simulink model "pwm_dc_control"  (R2022a)
settings: Solver=VariableStepAuto  StartTime=0.0  StopTime=4  RelTol=1e-3
model workspace (MATLAB code in the model file):
  | R = 1.71;
  | L = 1.1*10^-4;
  | kT = 5.9*10^-3;
  | kB = 2.75*10^-4;
  | I = 3.88*10^-7;
  | B = [0, -1/I; 1/L, 0];
  | A = [0, kT/I; -kB/L, -R/L];
  | C = [1, 0];
libraries: simulink x2
settings Model: Creator=ba13  LastModifiedBy=ba13
settings DataIOCC: Refine=100

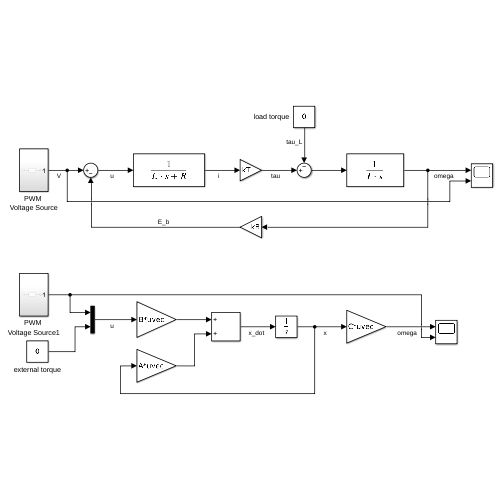
[thumbnail: Simulink's stored preview of the top-level diagram]
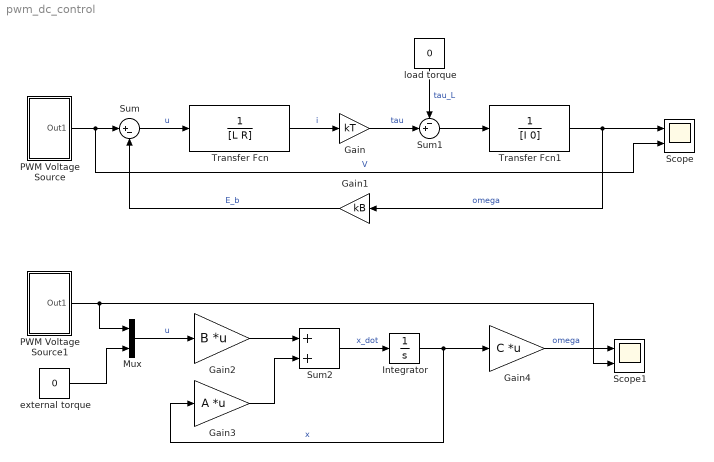
== system pwm_dc_control ==
  Gain : Gain  Gain=kT
  Gain1 : Gain  Gain=kB
  Gain2 : Gain  Gain=B  Multiplication=Matrix(K*u) (u vector)
  Gain3 : Gain  Gain=A  Multiplication=Matrix(K*u) (u vector)
  Gain4 : Gain  Gain=C  Multiplication=Matrix(K*u) (u vector)
  Integrator : Integrator
  Mux : Mux  Inputs=2
  PWM Voltage Source : Subsystem
  PWM Voltage Source1 : Subsystem
  Scope : Scope  NumInputPorts=2
  Scope1 : Scope  NumInputPorts=2
  Sum : Sum  Inputs=|+-
  Sum1 : Sum  Inputs=-+|
  Sum2 : Sum
  Transfer Fcn : TransferFcn  Denominator=[L R]
  Transfer Fcn1 : TransferFcn  Denominator=[I 0]
  external torque : Constant  Value=0
  load torque : Constant  Value=0
  wires:
  Sum/1 -> Transfer Fcn/1  "u"
  Transfer Fcn/1 -> Gain/1  "i"
  Gain/1 -> Sum1/2  "tau"
  Sum1/1 -> Transfer Fcn1/1
  Transfer Fcn1/1 -> Gain1/1, Scope/1  "omega"
  Gain1/1 -> Sum/2  "E_b"
  load torque/1 -> Sum1/1  "tau_L"
  PWM Voltage Source/1(Out1) -> Scope/2, Sum/1  "V"
  PWM Voltage Source1/1(Out1) -> Scope1/2, Mux/1
  external torque/1 -> Mux/2
  Mux/1 -> Gain2/1  "u"
  Gain2/1 -> Sum2/1
  Gain3/1 -> Sum2/2
  Sum2/1 -> Integrator/1  "x_dot"
  Integrator/1 -> Gain4/1, Gain3/1  "x"
  Gain4/1 -> Scope1/1  "omega"

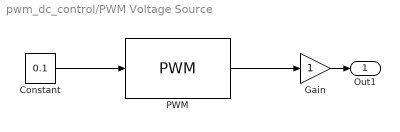
== system pwm_dc_control/PWM Voltage Source ==
  Constant : Constant  Value=0.1
  Gain : Gain
  PWM : simulink/Discontinuities/PWM  DisableCoverage=on  Period=0.001  DisallowZeroDutyCycle=off  RunAtFixedTimeIntervals=off  SampleTime=0.1
  Out1 : Outport
  wires:
  Constant/1 -> PWM/1
  PWM/1 -> Gain/1
  Gain/1 -> Out1/1

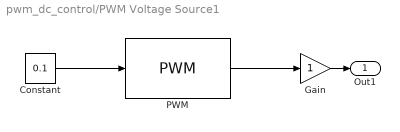
== system pwm_dc_control/PWM Voltage Source1 ==
  Constant : Constant  Value=0.1
  Gain : Gain
  PWM : simulink/Discontinuities/PWM  DisableCoverage=on  Period=0.001  DisallowZeroDutyCycle=off  RunAtFixedTimeIntervals=off  SampleTime=0.1
  Out1 : Outport
  wires:
  Gain/1 -> Out1/1
  PWM/1 -> Gain/1
  Constant/1 -> PWM/1
